simulink model "sofb"  (Simulink 7.8)
settings: Solver=ode45  StartTime=0.0  StopTime=10.0  RelTol=1e-3
values from neighbouring files (symbols this model uses):
  fofbctrl = param.fofbctrl    [simofb.m]
  sofbctrl = param.sofbctrl    [simofb.m]
libraries: cstblocks x2
settings Model: Creator=danielot  LastModifiedBy=danielot
settings OptimizationCC: InlineParams=on
settings DebuggingCC: ModelReferenceExtraNoncontSigs=none

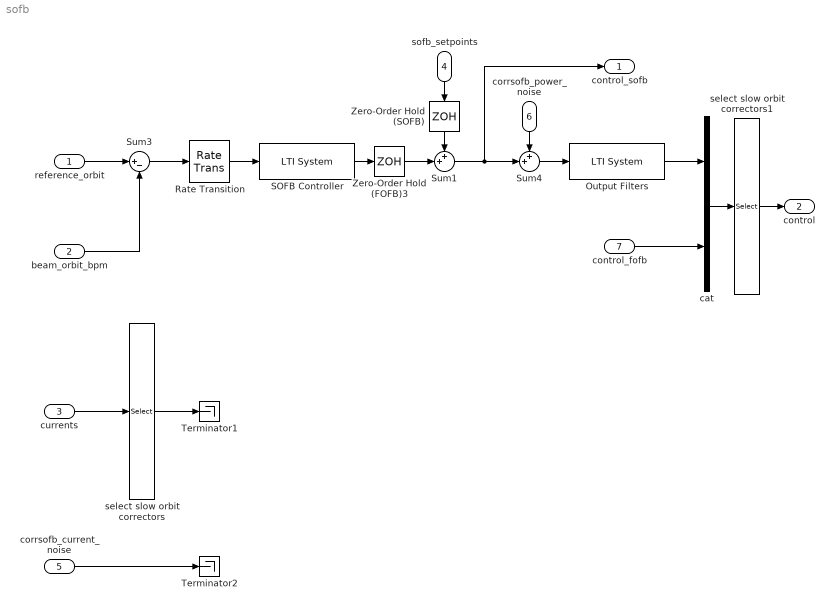
== system sofb ==
  reference_orbit : Inport  PortDimensions=nbpm
  beam_orbit_bpm : Inport  Port=2  PortDimensions=nbpm
  currents : Inport  Port=3  PortDimensions=ncorrmagnet
  sofb_setpoints : Inport  Port=4  PortDimensions=ncorrsofb
  corrsofb_current_noise : Inport  Port=5  PortDimensions=ncorrsofb
  corrsofb_power_noise : Inport  Port=6  PortDimensions=ncorrsofb
  control_fofb : Inport  Port=7  PortDimensions=ncorrfofb
  Output Filters : cstblocks/LTI System  sys=corrpsfilter  IC=[]
  Rate Transition : RateTransition  OutPortSampleTimeMultiple=ceil(fofbctrl.Ts/sofbctrl.Ts)
  SOFB Controller : cstblocks/LTI System  sys=sofbctrl  IC=[]
  Sum1 : Sum  Inputs=++|
  Sum3 : Sum  Inputs=|+-
  Sum4 : Sum  Inputs=++|  SampleTime=sofbctrl.Ts
  Terminator1 : Terminator
  Terminator2 : Terminator
  Zero-Order Hold (FOFB)3 : ZeroOrderHold  SampleTime=sofbctrl.Ts
  Zero-Order Hold (SOFB) : ZeroOrderHold  SampleTime=sofbctrl.Ts
  cat : Concatenate  Mode=Vector
  select slow orbit correctors : Selector  InputPortWidth=ncorrmagnet  IndexOptions=Index vector (dialog)  Indices=corrsofbselect  OutputSizes=1
  select slow orbit correctors1 : Selector  InputPortWidth=ncorr  IndexOptions=Index vector (dialog)  Indices=corrordering  OutputSizes=1
  control_sofb : Outport
  control : Outport  Port=2
  wires:
  cat/1 -> select slow orbit correctors1/1
  Output Filters/1 -> cat/1
  SOFB Controller/1 -> Zero-Order Hold (FOFB)3/1
  Rate Transition/1 -> SOFB Controller/1
  Zero-Order Hold (FOFB)3/1 -> Sum1/2
  Zero-Order Hold (SOFB)/1 -> Sum1/1
  sofb_setpoints/1 -> Zero-Order Hold (SOFB)/1
  Sum1/1 -> control_sofb/1, Sum4/2
  currents/1 -> select slow orbit correctors/1
  control_fofb/1 -> cat/2
  select slow orbit correctors1/1 -> control/1
  Sum4/1 -> Output Filters/1
  select slow orbit correctors/1 -> Terminator1/1
  beam_orbit_bpm/1 -> Sum3/2
  reference_orbit/1 -> Sum3/1
  Sum3/1 -> Rate Transition/1
  corrsofb_power_noise/1 -> Sum4/1
  corrsofb_current_noise/1 -> Terminator2/1
